simulink model "rectangular"  (Simulink 6.6)
settings: Solver=VariableStepDiscrete  StartTime=0.0  StopTime=1000  RelTol=1e-3
PreLoadFcn:
  | Fs = 1;
StopFcn:
  | samples = [1:20:981];
  | sample_vec = zeros(1,1000);
  | sample_vec(samples) = 1;
  | 
  | figure(1)
  | subplot(3,1,1)
  | plot(tx_signal,'m');
  | legend('Transmitted',4);
  | axis([0 length(tx_signal) -1.2 1.2]);
  | xlabel('Samples');
  | ylabel('Amplitude');
  | subplot(3,1,2)
  | hold off
  | plot([0 length(rx_signal)],[0 0],'k--');
  | hold on
  | plot(rx_signal,'b');
  | legend('Decision Line!','Received',1);
  | axis([0 length(rx_signal) 1.2*min(rx_signal) 1.2*max(rx_signal)]);
  | xlabel('Samples');
  | ylabel('Amplitude');
  | subplot(3,1,3)
  | hold off
  | plot(mf_signal,'r');
  | hold on
  | plot(sample_vec,'k');
  | legend('Matched Filtered', 'Max Effect Points',4);
  | axis([0 length(mf_signal) 1.2*min(mf_signal) 1.2*max(mf_signal)]);
  | xlabel('Samples');
  | ylabel('Amplitude');
undefined symbols (not defined in the file): dfilt
libraries: xbsIndex_r4 x4, dspsrcs4 x1, dsparch4 x1, dspsigops x1
settings Model: Creator=lcrockett  LastModifiedBy=lcrockett

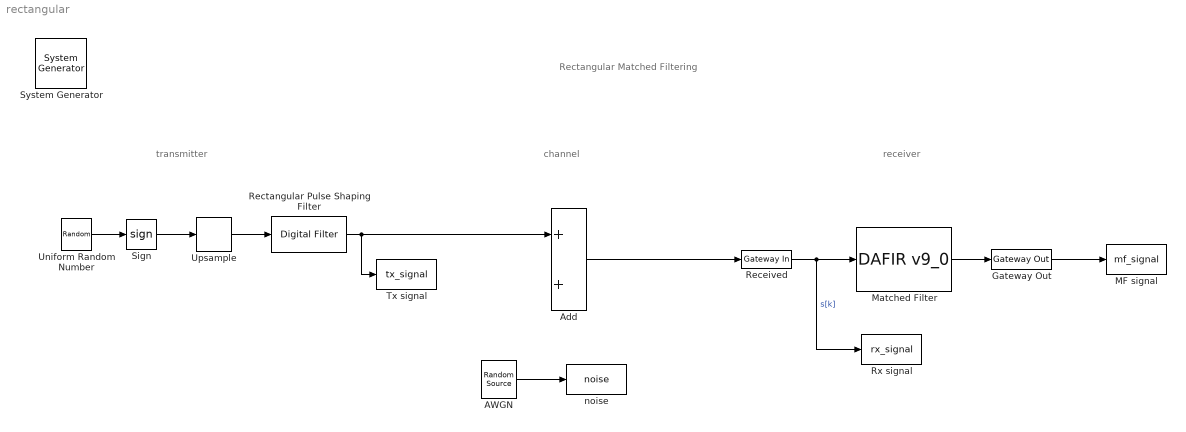
== system rectangular ==
  note: Rectangular Matched Filtering
  note: transmitter
  note: channel
  note: receiver
  " System Generator" : xbsIndex_r4/ System Generator  Tag=genX  SystemSampleTime=-1  xilinxfamily=virtex4  part=xc4vsx35  speed=-10  package=ff668  synthesis_tool=XST  clock_wrapper=Clock Enables  directory=./netlist  testbench=off  simulink_period=1/Fs  sysclk_period=10  dcm_input_clock_period=100  incr_netlist=off  trim_vbits=Everywhere in SubSystem  dbl_ovrd=According to Block Masks  core_generation=According to Block Masks  run_coregen=off  deprecated_control=off  eval_field=0  block_type=sysgen
      settings: block_version=9.2.01
  AWGN : dspsrcs4/Random Source  SrcType=Gaussian  NormMethod=Ziggurat  CltLength=12  MinVal=0  MaxVal=1  MeanVal=0  VarVal=0.4  RepMode=Not repeatable  rawSeed=1  IsInherit=on  SampMode=Discrete  SampTime=1  SampFrame=1  DataType=Single  OutComplex=Real
  Add : Sum  OutDataTypeMode=double  OutScaling=2^-10
  Gateway Out : xbsIndex_r4/Gateway Out  hdl_port=on  timing_constraint=None  locs_specified=off  LOCs={}  block_type=gatewayout
      settings: infoedit="Gateway out block.  Converts Xilinx fixed point inputs into ouputs of type Simulink integer, double, or fixed point.<P><P>Hardware notes:  In hardware these blocks become top level output ports or are discarded, depending on how they are configured."  block_version=10.1
  MF signal : ToWorkspace  VariableName=mf_signal  SampleTime=1  SaveFormat=Array
  "Matched Filter " : xbsIndex_r4/DAFIR v9_0   coef=(1/20)*ones(1,20)  structure=Inferred from Coefficients  coef_n_bits=16  coef_bin_pt=14  over_sample=1  reload=off  valids=off  rst=off  latency=1  num_channels=1  serial_input=off  polyphase_behavior="Single Rate:  sample in - sample out"  dbl_ovrd=off  explicit_period=off  period=1  use_isim=0  block_type=fir
      settings: infoedit="Hardware notes: Implemented using distributed arithmetic (DA).  The hardware over sampling rate determines the degree of parallelism.  A rate of one produces a fully parallel DA filter.  A rate of n (resp., n+1) for an n-bit input signal produces a fully serial implementation for a non-symmetric (resp., symmetric) impulse response.  Intermediate values produce implementations with intermediate levels of parallelism."  block_version=9.2.01
  Received : xbsIndex_r4/Gateway In  arith_type="Signed  (2's comp)"  n_bits=20  bin_pt=14  quantization="Round  (unbiased: +/- Inf)"  overflow=Saturate  period=1/Fs  dbl_ovrd=off  timing_constraint=None  locs_specified=off  LOCs={}  block_type=gatewayin
      settings: infoedit="Gateway in block.  Converts inputs of type Simulink integer, double and fixed point to  Xilinx fixed point type.<P><P>Hardware notes:  In hardware these blocks become top level input ports."  block_version=9.2.01
  Rectangular Pulse Shaping Filter : dsparch4/Digital Filter  DialogController=dspdialog.DigitalFilter  DialogControllerArgs=DataTag2  TypePopup=FIR (all zeros)  IIRFiltStruct=Direct form II transposed  AllPoleFiltStruct=Direct form  FIRFiltStruct=Direct form  CoeffSource=Specify via dialog  NumCoeffs=ones(1,20)  DenCoeffs=[1 0.1]  BiQuadCoeffs=[1 0.3 0.4 1 0.1 0.2]  LatticeCoeffs=[0.2 0.4]  denIgnore=on  FiltPerSampPopup=One filter per frame  IC=0  ICnum=0  ICden=0  roundingMode=Floor  overflowMode=off  ScaleValues=1  scaleValueFracLength=14  stageInFracLength=15  stageOutFracLength=15  FilterSource=Specify via dialog  dfiltObjectName=dfilt.dffir([1 2 1])
  Rx signal : ToWorkspace  VariableName=rx_signal  SampleTime=1  SaveFormat=Array
  Sign : Signum
  Tx signal : ToWorkspace  VariableName=tx_signal  SampleTime=1  SaveFormat=Array
  Uniform Random Number : UniformRandomNumber  Seed=rand(1,1)  SampleTime=20
  Upsample : dspsigops/Upsample  N=20  phase=0  ic=0  mode=Maintain input frame size
  noise : ToWorkspace  VariableName=noise  SampleTime=1  SaveFormat=Array
  wires:
  Received/1 -> "Matched Filter "/1, Rx signal/1  "s[k]"
  Uniform Random Number/1 -> Sign/1
  Sign/1 -> Upsample/1
  Upsample/1 -> Rectangular Pulse Shaping Filter/1
  Add/1 -> Received/1
  Rectangular Pulse Shaping Filter/1 -> Add/1, Tx signal/1
  AWGN/1 -> noise/1
  "Matched Filter "/1 -> Gateway Out/1
  Gateway Out/1 -> MF signal/1
